simulink model "flightControlSystem"  (R2020a)
settings: Solver=ode3  StartTime=0  StopTime=TFinal  FixedStep=Ts  RelTol=1e-3  EnableMultiTasking=on
undefined symbols (not defined in the file): codertarget, Controller, DiscIntNeverNeededParam, Discrete, Estimator, g, gray, init, orient_ref, pos_ref, Sensors, Time, Ts, Vehicle
libraries: simulink x37, sharedtransform x3, ctrlSharedLib x2, visionstatistics x2, visiontransforms x2, sharedutil x1, visiontextngfix x1, visionanalysis x1, parrotlib x1
(part 2 of 2)

== system flightControlSystem/Control System/State Estimator/EstimatorXYPosition ==
  opticalFlow_datin : Inport
  controlModePosVSOrient_flagin : Inport  Port=2
  sensorIMU_datin : Inport  Port=3
  Z_estimin : Inport  Port=4
  dz_estimin : Inport  Port=5
  orient_estimin : Inport  Port=6
  EstimatorVelocity : Subsystem
  EstimatorXYPosition : Subsystem
  XY_estimout : Outport  VectorParamsAs1DForOutWhenUnconnected=off
  dxy_estimout : Outport  Port=2  VectorParamsAs1DForOutWhenUnconnected=off
  wires:
  EstimatorXYPosition/1(XY_estimout) -> XY_estimout/1
  dz_estimin/1 -> EstimatorXYPosition/4(dz_estimin)
  controlModePosVSOrient_flagin/1 -> EstimatorXYPosition/3(controlModePosVSOrient_flagin)
  Z_estimin/1 -> EstimatorVelocity/2(Z_estimin)
  sensorIMU_datin/1 -> EstimatorVelocity/3(sensorIMU_datin)
  opticalFlow_datin/1 -> EstimatorVelocity/1(opticalFlow_datin)
  EstimatorVelocity/1(dxy_estimout) -> dxy_estimout/1, EstimatorXYPosition/1(dxy_estimin)
  orient_estimin/1 -> EstimatorVelocity/4(orient_estimin), EstimatorXYPosition/2(orient_estimin)

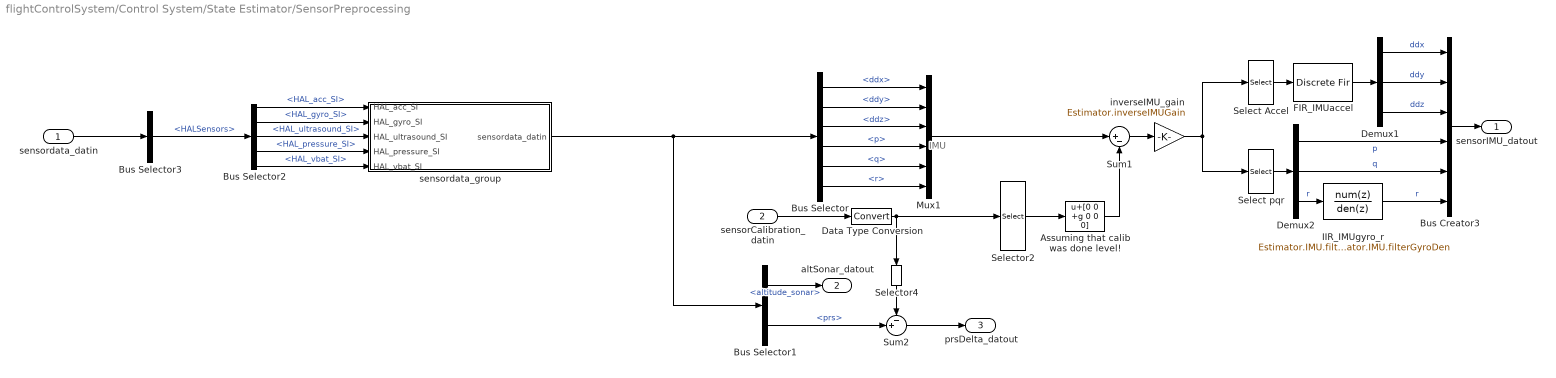
== system flightControlSystem/Control System/State Estimator/SensorPreprocessing ==
  note: IMU
  sensordata_datin : Inport
  sensorCalibration_datin : Inport  Port=2
  Assuming that calib was done level! : Bias  Bias=[0 0 +g 0 0 0]
  Bus Creator3 : BusCreator  Inputs=6
  Bus Selector : BusSelector  OutputSignals=ddx,ddy,ddz,p,q,r
  Bus Selector1 : BusSelector  OutputSignals=altitude_sonar,prs
  Bus Selector2 : BusSelector  OutputSignals=HAL_acc_SI,HAL_gyro_SI,HAL_ultrasound_SI,HAL_pressure_SI,HAL_vbat_SI
  Bus Selector3 : BusSelector  OutputSignals=HALSensors
  Data Type Conversion : DataTypeConversion
  Demux1 : Demux  Outputs=3
  Demux2 : Demux  Outputs=3
  FIR_IMUaccel : DiscreteFir  Coefficients=Estimator.IMU.filterAccel.Coefficients
  IIR_IMUgyro_r : DiscreteFilter  Numerator=Estimator.IMU.filterGyroNum  Denominator=Estimator.IMU.filterGyroDen
  Mux1 : Mux  Inputs=6
  Select Accel : Selector  InputPortWidth=6  IndexOptions=Index vector (dialog)  Indices=[1 2 3]  OutputSizes=1
  Select pqr : Selector  InputPortWidth=6  IndexOptions=Index vector (dialog)  Indices=[4 5 6]  OutputSizes=1
  Selector2 : Selector  InputPortWidth=8  IndexOptions=Index vector (dialog)  Indices=[1:6]  OutputSizes=1
  Selector4 : Selector  InputPortWidth=8  IndexOptions=Index vector (dialog)  Indices=[7]  OutputSizes=1
  Sum1 : Sum  Inputs=|+-
  Sum2 : Sum  Inputs=-+|
  inverseIMU_gain : Gain  Gain=Estimator.inverseIMUGain  ParamDataTypeStr=single  OutDataTypeStr=single
  sensordata_group : Subsystem
  sensorIMU_datout : Outport  VectorParamsAs1DForOutWhenUnconnected=off
  altSonar_datout : Outport  Port=2  VectorParamsAs1DForOutWhenUnconnected=off
  prsDelta_datout : Outport  Port=3  VectorParamsAs1DForOutWhenUnconnected=off
  wires:
  Select pqr/1 -> Demux2/1
  Assuming that calib was done level!/1 -> Sum1/2
  Mux1/1 -> Sum1/1
  Sum2/1 -> prsDelta_datout/1
  Bus Selector1/2 -> Sum2/2  "<prs>"
  Selector4/1 -> Sum2/1
  Bus Selector1/1 -> altSonar_datout/1  "<altitude_sonar>"
  Bus Selector/6 -> Mux1/6  "<r>"
  Bus Selector/5 -> Mux1/5  "<q>"
  Bus Selector/4 -> Mux1/4  "<p>"
  Bus Selector/3 -> Mux1/3  "<ddz>"
  Bus Selector/2 -> Mux1/2  "<ddy>"
  Bus Selector/1 -> Mux1/1  "<ddx>"
  sensorCalibration_datin/1 -> Data Type Conversion/1
  IIR_IMUgyro_r/1 -> Bus Creator3/6  "r"
  Demux2/3 -> IIR_IMUgyro_r/1  "r"
  FIR_IMUaccel/1 -> Demux1/1
  Select Accel/1 -> FIR_IMUaccel/1
  inverseIMU_gain/1 -> Select Accel/1, Select pqr/1
  Demux2/2 -> Bus Creator3/5  "q"
  Demux2/1 -> Bus Creator3/4  "p"
  Selector2/1 -> Assuming that calib was done level!/1
  Sum1/1 -> inverseIMU_gain/1
  Demux1/3 -> Bus Creator3/3  "ddz"
  Demux1/2 -> Bus Creator3/2  "ddy"
  Demux1/1 -> Bus Creator3/1  "ddx"
  Bus Creator3/1 -> sensorIMU_datout/1
  Data Type Conversion/1 -> Selector2/1, Selector4/1
  Bus Selector2/2 -> sensordata_group/2(HAL_gyro_SI)  "<HAL_gyro_SI>"
  Bus Selector2/4 -> sensordata_group/4(HAL_pressure_SI)  "<HAL_pressure_SI>"
  Bus Selector2/5 -> sensordata_group/5(HAL_vbat_SI)  "<HAL_vbat_SI>"
  Bus Selector2/3 -> sensordata_group/3(HAL_ultrasound_SI)  "<HAL_ultrasound_SI>"
  Bus Selector3/1 -> Bus Selector2/1  "<HALSensors>"
  sensordata_group/1(sensordata_datin) -> Bus Selector1/1, Bus Selector/1
  sensordata_datin/1 -> Bus Selector3/1
  Bus Selector2/1 -> sensordata_group/1(HAL_acc_SI)  "<HAL_acc_SI>"

== system flightControlSystem/Control System/State Estimator/Complementary Filter/If Action Subsystem ==
  rpy : Inport
  accel : Inport  Port=2
  Action Port : ActionPort  ActionPortLabel=if(u1 > 0)
  Demux : Demux  Outputs=3
  Demux1 : Demux  Outputs=3
  Divide : Product  Inputs=*/
  Gain : Gain  Gain=1-Estimator.gyroAngleUpdateAccWeight
  Gain1 : Gain  Gain=Estimator.gyroAngleUpdateAccWeight
  Gain2 : Gain  Gain=1/g
  Gain3 : Gain  Gain=Estimator.gyroAngleUpdateAccWeight
  Gain4 : Gain  Gain=1-Estimator.gyroAngleUpdateAccWeight
  Mux : Mux  Inputs=2
  Sum : Sum  Inputs=|++
  Sum1 : Sum  Inputs=|++
  Terminator1 : Terminator
  Trigonometric Function : Trigonometry  Operator=atan
  Trigonometric Function1 : Trigonometry  Operator=asin
  pitch,roll : Outport  VectorParamsAs1DForOutWhenUnconnected=off
  wires:
  accel/1 -> Demux/1
  Demux/2 -> Divide/1
  Demux/3 -> Divide/2
  Divide/1 -> Trigonometric Function/1
  Gain/1 -> Sum/1
  Trigonometric Function/1 -> Gain1/1
  Mux/1 -> pitch,roll/1
  Gain2/1 -> Trigonometric Function1/1
  Trigonometric Function1/1 -> Gain3/1
  Gain4/1 -> Sum1/1
  Gain3/1 -> Sum1/2
  Sum1/1 -> Mux/1
  Sum/1 -> Mux/2
  rpy/1 -> Demux1/1
  Demux1/1 -> Gain/1
  Demux1/2 -> Gain4/1
  Demux/1 -> Gain2/1
  Demux1/3 -> Terminator1/1
  Gain1/1 -> Sum/2

== system flightControlSystem/Control System/State Estimator/Complementary Filter/If Action Subsystem2 ==
  prin : Inport
  Action Port : ActionPort  ActionPortLabel=else
  prout : Outport  VectorParamsAs1DForOutWhenUnconnected=off
  wires:
  prin/1 -> prout/1

== system flightControlSystem/Control System/State Estimator/Complementary Filter/Wbe ==
  rpy : Inport  OutDataTypeStr=single
  Constant : Constant  Value=single(0)
  Create 3x3 Matrix : sharedutil/Create 3x3 Matrix  aMode=aMode
      settings: SourceProductBaseCode=AE,PW,MT,VE,VP
  Divide : Product  Inputs=*/
  Gain : Gain  Gain=-1
  Product{1..4} (4 alike) : Product
  Selector : Selector  InputPortWidth=3  IndexOptions=Index vector (dialog)  Indices=[1]  OutputSizes=1
  Selector1 : Selector  InputPortWidth=3  IndexOptions=Index vector (dialog)  Indices=[1]  OutputSizes=1
  Selector2 : Selector  InputPortWidth=3  IndexOptions=Index vector (dialog)  Indices=[2]  OutputSizes=1
  Selector3 : Selector  InputPortWidth=3  IndexOptions=Index vector (dialog)  Indices=[2]  OutputSizes=1
  Trigonometric Function : Trigonometry  Operator=sincos
  Wbe : Outport  VectorParamsAs1DForOutWhenUnconnected=off
  wires:
  Create 3x3 Matrix/1 -> Divide/1
  Product3/1 -> Create 3x3 Matrix/8
  Trigonometric Function/2 -> Selector1/1, Selector2/1
  Selector3/1 -> Product4/2, Product3/2
  Selector1/1 -> Product4/1, Product1/1, Create 3x3 Matrix/3
  Trigonometric Function/1 -> Selector3/1, Selector/1
  Product1/1 -> Create 3x3 Matrix/5
  Product2/1 -> Create 3x3 Matrix/6
  Selector2/1 -> Divide/2, Create 3x3 Matrix/7, Product2/1, Product1/2
  Gain/1 -> Product2/2
  Product4/1 -> Create 3x3 Matrix/9
  Constant/1 -> Create 3x3 Matrix/4, Create 3x3 Matrix/1
  Divide/1 -> Wbe/1
  rpy/1 -> Trigonometric Function/1
  Selector/1 -> Product3/1, Gain/1, Create 3x3 Matrix/2

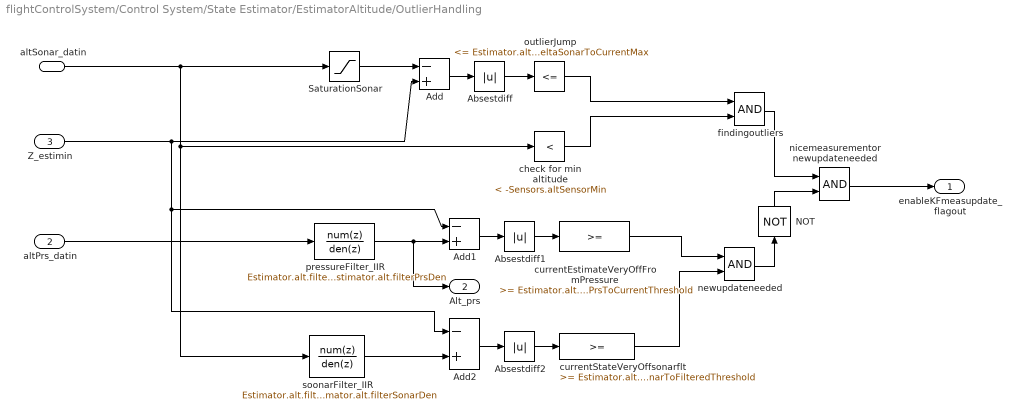
== system flightControlSystem/Control System/State Estimator/EstimatorAltitude/OutlierHandling ==
  altSonar_datin : Inport
  altPrs_datin : Inport  Port=2
  Z_estimin : Inport  Port=3
  Absestdiff : Abs
  Absestdiff1 : Abs
  Absestdiff2 : Abs
  Add : Sum  Inputs=-+
  Add1 : Sum  Inputs=-+
  Add2 : Sum  Inputs=-+
  NOT : Logic  Operator=NOT  IconShape=distinctive  AllPortsSameDT=off  OutDataTypeStr=boolean
  SaturationSonar : Saturate  UpperLimit=-Sensors.altSensorMin  LowerLimit=-inf
  check for min altitude : simulink/Logic and Bit Operations/Compare To Constant  relop=<  const=-Sensors.altSensorMin  OutDataTypeStr=boolean
  currentEstimateVeryOffFromPressure : simulink/Logic and Bit Operations/Compare To Constant  relop=>=  const=Estimator.alt.deltaPrsToCurrentThreshold  OutDataTypeStr=boolean
  currentStateVeryOffsonarflt : simulink/Logic and Bit Operations/Compare To Constant  relop=>=  const=Estimator.alt.deltaSonarToFilteredThreshold  OutDataTypeStr=boolean
  findingoutliers : Logic  AllPortsSameDT=off  OutDataTypeStr=boolean
  newupdateneeded : Logic  AllPortsSameDT=off  OutDataTypeStr=boolean
  nicemeasurementor newupdateneeded : Logic  AllPortsSameDT=off  OutDataTypeStr=boolean
  outlierJump : simulink/Logic and Bit Operations/Compare To Constant  relop=<=  const=Estimator.alt.deltaSonarToCurrentMax  OutDataTypeStr=boolean
  pressureFilter_IIR : DiscreteFilter  Numerator=Estimator.alt.filterPrsNum  Denominator=Estimator.alt.filterPrsDen
  soonarFilter_IIR : DiscreteFilter  Numerator=Estimator.alt.filterSonarNum  Denominator=Estimator.alt.filterSonarDen
  enableKFmeasupdate_flagout : Outport  VectorParamsAs1DForOutWhenUnconnected=off
  Alt_prs : Outport  Port=2  VectorParamsAs1DForOutWhenUnconnected=off
  wires:
  Add1/1 -> Absestdiff1/1
  nicemeasurementor newupdateneeded/1 -> enableKFmeasupdate_flagout/1
  findingoutliers/1 -> nicemeasurementor newupdateneeded/1
  check for min altitude/1 -> findingoutliers/2
  outlierJump/1 -> findingoutliers/1
  SaturationSonar/1 -> Add/1
  Absestdiff/1 -> outlierJump/1
  Add/1 -> Absestdiff/1
  newupdateneeded/1 -> NOT/1
  Absestdiff2/1 -> currentStateVeryOffsonarflt/1
  altSonar_datin/1 -> SaturationSonar/1, soonarFilter_IIR/1, check for min altitude/1
  currentEstimateVeryOffFromPressure/1 -> newupdateneeded/1
  Z_estimin/1 -> Add1/1, Add2/1, Add/2
  Add2/1 -> Absestdiff2/1
  currentStateVeryOffsonarflt/1 -> newupdateneeded/2
  pressureFilter_IIR/1 -> Alt_prs/1, Add1/2
  altPrs_datin/1 -> pressureFilter_IIR/1
  soonarFilter_IIR/1 -> Add2/2
  Absestdiff1/1 -> currentEstimateVeryOffFromPressure/1
  NOT/1 -> nicemeasurementor newupdateneeded/2

== system flightControlSystem/Control System/State Estimator/EstimatorXYPosition/EstimatorVelocity ==
  opticalFlow_datin : Inport
  Z_estimin : Inport  Port=2  SampleTime=Ts
  sensorIMU_datin : Inport  Port=3
  orient_estimin : Inport  Port=4
  " " : Product  Inputs=**
  AccelerationHandling : Subsystem
  Compare To Constant : simulink/Logic and Bit Operations/Compare To Constant  relop=<  const=200*4  OutDataTypeStr=boolean
  Counter Free-Running : simulink/Sources/Counter Free-Running  NumBits=32  tsamp=-1
  DataHandling : Subsystem
  Delay : Delay  DelayLength=1  InitialCondition=0
  Gain : Gain  Gain=-1
  KalmanFilter_dxdy : ctrlSharedLib/Kalman Filter  TimeDomain=Discrete-Time  UseCurrentEstimator=on  ModelSource=Individual A, B, C, D matrices  ModelSourceVariable=ss(0.95,1,1,0,1)  A=eye(2)  B=Ts*eye(2)  C=eye(2)  D=0  NumberOfStates=1  NumberOfInputs=1  NumberOfOutputs=1  InitialEstimateSource=Dialog  X0=0  P0=10  UseK=off  UseGH=on  NumberOfProcessNoiseInputs=1  G=Estimator.pos.kfVelo.G  TimeInvariantG=on  H=Estimator.pos.kfVelo.H  TimeInvariantH=on  Q=Estimator.pos.kfVelo.Q  TimeInvariantQ=on  R=Estimator.pos.kfVelo.R  TimeInvariantR=on  N=Estimator.pos.kfVelo.N  TimeInvariantN=on  AddInputPort=on  AddEnablePort=on  OutputEstimatedY=off  OutputP=off  Ts=-1
  Select dxy : Selector  InputPortWidth=3  IndexOptions=Index vector (dialog)  Indices=[1 2]  OutputSizes=1
  Switch : Switch  Criteria=u2 > Threshold
  Z_estimin1 : InportShadow  Port=2  SampleTime=Ts
  opticalFlowErrorCorrect : Gain  Gain=1.15
  dxy_estimout : Outport  VectorParamsAs1DForOutWhenUnconnected=off
  wires:
  Delay/1 -> DataHandling/5(dxyOF_datin)
  Z_estimin/1 -> DataHandling/1(Z_estimin), AccelerationHandling/4(Z_estimin)
  KalmanFilter_dxdy/1 -> dxy_estimout/1, Delay/1
  sensorIMU_datin/1 -> AccelerationHandling/2(sensorIMU_datin), DataHandling/3(sensorIMU_datin)
  orient_estimin/1 -> AccelerationHandling/3(orient_estimin), DataHandling/2(orient_estimin)
  Select dxy/1 -> KalmanFilter_dxdy/2, AccelerationHandling/1(dxy_estimin), DataHandling/4(dxy_estimin)
  AccelerationHandling/1(acceleration_world) -> KalmanFilter_dxdy/1
  DataHandling/1(enable_flag) -> KalmanFilter_dxdy/3
  Switch/1 -> Select dxy/1
  " "/1 -> opticalFlowErrorCorrect/1
  Gain/1 -> " "/2
  opticalFlowErrorCorrect/1 -> Switch/3
  Compare To Constant/1 -> Switch/2
  opticalFlow_datin/1 -> " "/1, Switch/1
  Z_estimin1/1 -> Gain/1
  Counter Free-Running/1 -> Compare To Constant/1

== system flightControlSystem/Control System/State Estimator/EstimatorXYPosition/EstimatorXYPosition ==
  note: Switching from orientationControl to Position
      | control reset the current world position estimate
      | (happens when using no markers)
  dxy_estimin : Inport
  orient_estimin : Inport  Port=2  SampleTime=Ts
  controlModePosVSOrient_flagin : Inport  Port=3
  dz_estimin : Inport  Port=4
  Math Function : Math  Operator=transpose  SignedPower=on  SaturateOnIntegerOverflow=on
  Mux2 : Mux  Inputs=2
  Product : Product  Multiplication=Matrix(*)
  Rotation Angles to Direction Cosine Matrix : sharedtransform/Rotation Angles to Direction Cosine Matrix  rotationOrder=ZYX  aMode=aMode
      settings: SourceProductBaseCode=AE,PW,MT,VE,VP
  SelectdXY : Selector  InputPortWidth=3  IndexOptions=Index vector (dialog)  Indices=[1 2]  OutputSizes=1
  SimplyIntegrateVelocity : DiscreteIntegrator  ExternalReset=rising  SampleTime=Ts  ICPrevOutput=DiscIntNeverNeededParam  ICPrevScaledInput=DiscIntNeverNeededParam
  XY_estimout : Outport  VectorParamsAs1DForOutWhenUnconnected=off
  wires:
  controlModePosVSOrient_flagin/1 -> SimplyIntegrateVelocity/2
  Product/1 -> SelectdXY/1
  Mux2/1 -> Product/2
  dz_estimin/1 -> Mux2/2
  SimplyIntegrateVelocity/1 -> XY_estimout/1
  dxy_estimin/1 -> Mux2/1
  orient_estimin/1 -> Rotation Angles to Direction Cosine Matrix/1
  Rotation Angles to Direction Cosine Matrix/1 -> Math Function/1
  SelectdXY/1 -> SimplyIntegrateVelocity/1
  Math Function/1 -> Product/1

== system flightControlSystem/Control System/State Estimator/SensorPreprocessing/sensordata_group ==
  HAL_acc_SI : Inport  OutDataTypeStr=Bus: HAL_acc_SI_t
  HAL_gyro_SI : Inport  Port=2  OutDataTypeStr=Bus: HAL_gyro_SI_t
  HAL_ultrasound_SI : Inport  Port=3  OutDataTypeStr=Bus: HAL_ultrasound_SI_t
  HAL_pressure_SI : Inport  Port=4  OutDataTypeStr=Bus: HAL_pressure_SI_t
  HAL_vbat_SI : Inport  Port=5  OutDataTypeStr=Bus: HAL_vbat_SI_t
  Bus Selector1 : BusSelector  OutputSignals=vbat_V,vbat_percentage
  Bus Selector3 : BusSelector  OutputSignals=x,y,z
  Bus Selector4 : BusSelector  OutputSignals=x,y,z
  Bus Selector5 : BusSelector  OutputSignals=altitude
  Bus Selector6 : BusSelector  OutputSignals=pressure
  Out Bus Element : Outport  VectorParamsAs1DForOutWhenUnconnected=off  PortName=sensordata_datin  Element=ddx
  Out Bus Element1 : Outport  VectorParamsAs1DForOutWhenUnconnected=off  PortName=sensordata_datin  Element=ddy
  Out Bus Element2 : Outport  VectorParamsAs1DForOutWhenUnconnected=off  PortName=sensordata_datin  Element=ddz
  Out Bus Element3 : Outport  VectorParamsAs1DForOutWhenUnconnected=off  PortName=sensordata_datin  Element=p
  Out Bus Element4 : Outport  VectorParamsAs1DForOutWhenUnconnected=off  PortName=sensordata_datin  Element=q
  Out Bus Element5 : Outport  VectorParamsAs1DForOutWhenUnconnected=off  PortName=sensordata_datin  Element=r
  Out Bus Element6 : Outport  VectorParamsAs1DForOutWhenUnconnected=off  PortName=sensordata_datin  Element=altitude_sonar
  Out Bus Element7 : Outport  VectorParamsAs1DForOutWhenUnconnected=off  PortName=sensordata_datin  Element=prs
  Out Bus Element8 : Outport  VectorParamsAs1DForOutWhenUnconnected=off  PortName=sensordata_datin  Element=vbat_V
  Out Bus Element9 : Outport  VectorParamsAs1DForOutWhenUnconnected=off  PortName=sensordata_datin  Element=vbat_percentage
  wires:
  HAL_gyro_SI/1 -> Bus Selector4/1
  HAL_acc_SI/1 -> Bus Selector3/1
  HAL_pressure_SI/1 -> Bus Selector6/1
  HAL_ultrasound_SI/1 -> Bus Selector5/1
  Bus Selector4/1 -> Out Bus Element3/1  "<x>"
  Bus Selector3/3 -> Out Bus Element2/1  "<z>"
  Bus Selector4/3 -> Out Bus Element5/1  "<z>"
  Bus Selector5/1 -> Out Bus Element6/1  "<altitude>"
  Bus Selector6/1 -> Out Bus Element7/1  "<pressure>"
  Bus Selector4/2 -> Out Bus Element4/1  "<y>"
  Bus Selector3/1 -> Out Bus Element/1  "<x>"
  Bus Selector3/2 -> Out Bus Element1/1  "<y>"
  Bus Selector1/1 -> Out Bus Element8/1  "<vbat_V>"
  HAL_vbat_SI/1 -> Bus Selector1/1
  Bus Selector1/2 -> Out Bus Element9/1  "<vbat_percentage>"

== system flightControlSystem/Control System/State Estimator/EstimatorXYPosition/EstimatorVelocity/AccelerationHandling ==
  dxy_estimin : Inport
  sensorIMU_datin : Inport  Port=2
  orient_estimin : Inport  Port=3
  Z_estimin : Inport  Port=4
  Add : Sum  Inputs=-+
  Bus Selector1 : BusSelector  OutputSignals=ddx,ddy,ddz
  Deactivate Acceleration If OF is not used due to low altitude : simulink/Logic and Bit Operations/Compare To Constant  relop=<=  const=Estimator.pos.opticalFlowZMax  OutDataTypeStr=boolean
  Logical Operator : Logic  Operator=OR  AllPortsSameDT=off  OutDataTypeStr=boolean
  Mux6 : Mux  Inputs=3
  Product : Product  Inputs=3
  Product1 : Product  Multiplication=Matrix(*)
  Rotation Angles to Direction Cosine Matrix : sharedtransform/Rotation Angles to Direction Cosine Matrix  rotationOrder=ZYX  aMode=aMode
      settings: SourceProductBaseCode=AE,PW,MT,VE,VP
  SelectPlanarddxy : Selector  InputPortWidth=3  IndexOptions=Index vector (dialog)  Indices=[1 2]  OutputSizes=1
  Selector : Selector  InputPortWidth=2  IndexOptions=Index vector (dialog)  Indices=1  OutputSizes=1
  Selector1 : Selector  InputPortWidth=2  IndexOptions=Index vector (dialog)  Indices=2  OutputSizes=1
  do not use acc if optical flow never available (Note OF@60Hz but ZOH to 200!) : simulink/Logic and Bit Operations/Compare To Constant  relop=~=  const=0  OutDataTypeStr=boolean
  do not use acc if optical flow never available (Note OF@60Hz but ZOH to 200!)1 : simulink/Logic and Bit Operations/Compare To Constant  relop=~=  const=0  OutDataTypeStr=boolean
  gainaccinput : Gain  Gain=Estimator.pos.accelerationInputGain  OutDataTypeStr=single
  gravity : Constant  Value=[0 0 -g]
  acceleration_world : Outport  OutDataTypeStr=single  VectorParamsAs1DForOutWhenUnconnected=off
  wires:
  do not use acc if optical flow never available (Note OF@60Hz but ZOH to 200!)1/1 -> Logical Operator/2
  do not use acc if optical flow never available (Note OF@60Hz but ZOH to 200!)/1 -> Logical Operator/1
  Logical Operator/1 -> Product/1
  Selector1/1 -> do not use acc if optical flow never available (Note OF@60Hz but ZOH to 200!)1/1
  Selector/1 -> do not use acc if optical flow never available (Note OF@60Hz but ZOH to 200!)/1
  dxy_estimin/1 -> Selector1/1, Selector/1
  Product/1 -> acceleration_world/1
  Deactivate Acceleration If OF is not used due to low altitude/1 -> Product/3
  Z_estimin/1 -> Deactivate Acceleration If OF is not used due to low altitude/1
  Add/1 -> SelectPlanarddxy/1
  Product1/1 -> Add/1
  gravity/1 -> Product1/2
  gainaccinput/1 -> Product/2
  SelectPlanarddxy/1 -> gainaccinput/1
  Bus Selector1/3 -> Mux6/3  "<ddz>"
  Bus Selector1/1 -> Mux6/1  "<ddx>"
  sensorIMU_datin/1 -> Bus Selector1/1
  Mux6/1 -> Add/2
  Bus Selector1/2 -> Mux6/2  "<ddy>"
  orient_estimin/1 -> Rotation Angles to Direction Cosine Matrix/1
  Rotation Angles to Direction Cosine Matrix/1 -> Product1/1

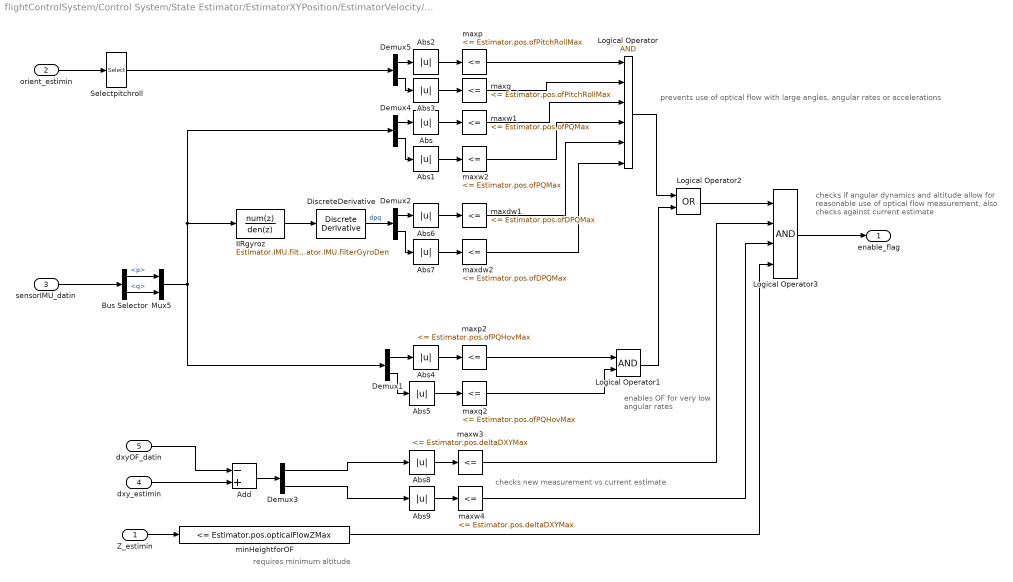
== system flightControlSystem/Control System/State Estimator/EstimatorXYPosition/EstimatorVelocity/DataHandling ==
  note: prevents use of optical flow with large angles, angular rates or accelerations
  note: enables OF for very
      | low angular rates
  note: checks if angular dynamics and altitude allow for
      | reasonable use of optical flow measurement,
      | also checks against current estimate
  note: checks new measurement vs current estimate
  note: requires minimum altitude
  Z_estimin : Inport
  orient_estimin : Inport  Port=2
  sensorIMU_datin : Inport  Port=3
  dxy_estimin : Inport  Port=4
  dxyOF_datin : Inport  Port=5
  Abs{,1..9} (10 alike) : Abs
  Add : Sum  Inputs=-+
  Bus Selector : BusSelector  OutputSignals=p,q
  Demux{1..5} (5 alike) : Demux  Outputs=2
  DiscreteDerivative : simulink/Discrete/Discrete Derivative  gainval=1.0  ICPrevScaledInput=0.0  OutMin=[]  OutMax=[]  OutDataType=fixdt(1, 16)  OutScaling=2^-10  DoSatur=off
  IIRgyroz : DiscreteFilter  Numerator=Estimator.IMU.filterGyroNum  Denominator=Estimator.IMU.filterGyroDen
  Logical Operator : Logic  Inputs=6  AllPortsSameDT=off  OutDataTypeStr=boolean
  Logical Operator1 : Logic  AllPortsSameDT=off  OutDataTypeStr=boolean
  Logical Operator2 : Logic  Operator=OR  AllPortsSameDT=off  OutDataTypeStr=boolean
  Logical Operator3 : Logic  Inputs=4  AllPortsSameDT=off  OutDataTypeStr=boolean
  Mux5 : Mux  Inputs=2
  Selectpitchroll : Selector  InputPortWidth=3  IndexOptions=Index vector (dialog)  Indices=[2 3]  OutputSizes=1
  maxdw1 : simulink/Logic and Bit Operations/Compare To Constant  relop=<=  const=Estimator.pos.ofDPQMax  OutDataTypeStr=boolean
  maxdw2 : simulink/Logic and Bit Operations/Compare To Constant  relop=<=  const=Estimator.pos.ofDPQMax  OutDataTypeStr=boolean
  maxp : simulink/Logic and Bit Operations/Compare To Constant  relop=<=  const=Estimator.pos.ofPitchRollMax  OutDataTypeStr=boolean
  maxp2 : simulink/Logic and Bit Operations/Compare To Constant  relop=<=  const=Estimator.pos.ofPQHovMax  OutDataTypeStr=boolean
  maxq : simulink/Logic and Bit Operations/Compare To Constant  relop=<=  const=Estimator.pos.ofPitchRollMax  OutDataTypeStr=boolean
  maxq2 : simulink/Logic and Bit Operations/Compare To Constant  relop=<=  const=Estimator.pos.ofPQHovMax  OutDataTypeStr=boolean
  maxw1 : simulink/Logic and Bit Operations/Compare To Constant  relop=<=  const=Estimator.pos.ofPQMax  OutDataTypeStr=boolean
  maxw2 : simulink/Logic and Bit Operations/Compare To Constant  relop=<=  const=Estimator.pos.ofPQMax  OutDataTypeStr=boolean
  maxw3 : simulink/Logic and Bit Operations/Compare To Constant  relop=<=  const=Estimator.pos.deltaDXYMax  OutDataTypeStr=boolean
  maxw4 : simulink/Logic and Bit Operations/Compare To Constant  relop=<=  const=Estimator.pos.deltaDXYMax  OutDataTypeStr=boolean
  minHeightforOF : simulink/Logic and Bit Operations/Compare To Constant  relop=<=  const=Estimator.pos.opticalFlowZMax  OutDataTypeStr=boolean
  enable_flag : Outport  VectorParamsAs1DForOutWhenUnconnected=off
  wires:
  minHeightforOF/1 -> Logical Operator3/4
  IIRgyroz/1 -> DiscreteDerivative/1
  Mux5/1 -> Demux1/1, IIRgyroz/1, Demux4/1
  maxw4/1 -> Logical Operator3/3
  maxw3/1 -> Logical Operator3/2
  dxyOF_datin/1 -> Add/1
  Demux3/2 -> Abs9/1
  Demux3/1 -> Abs8/1
  dxy_estimin/1 -> Add/2
  Add/1 -> Demux3/1
  Abs9/1 -> maxw4/1
  Abs8/1 -> maxw3/1
  Logical Operator2/1 -> Logical Operator3/1
  Logical Operator3/1 -> enable_flag/1
  DiscreteDerivative/1 -> Demux2/1  "dpq"
  Demux2/2 -> Abs7/1
  Demux2/1 -> Abs6/1
  Abs7/1 -> maxdw2/1
  Abs6/1 -> maxdw1/1
  Logical Operator1/1 -> Logical Operator2/2
  Demux1/2 -> Abs5/1
  Demux1/1 -> Abs4/1
  Abs5/1 -> maxq2/1
  Abs4/1 -> maxp2/1
  Abs3/1 -> maxq/1
  Abs2/1 -> maxp/1
  Demux4/2 -> Abs1/1
  Demux4/1 -> Abs/1
  Abs1/1 -> maxw2/1
  Abs/1 -> maxw1/1
  Z_estimin/1 -> minHeightforOF/1
  Logical Operator/1 -> Logical Operator2/1
  maxw1/1 -> Logical Operator/3
  Bus Selector/1 -> Mux5/1  "<p>"
  Selectpitchroll/1 -> Demux5/1
  sensorIMU_datin/1 -> Bus Selector/1
  maxq2/1 -> Logical Operator1/2
  Bus Selector/2 -> Mux5/2  "<q>"
  maxp/1 -> Logical Operator/1
  maxw2/1 -> Logical Operator/4
  orient_estimin/1 -> Selectpitchroll/1
  maxdw1/1 -> Logical Operator/5
  maxdw2/1 -> Logical Operator/6
  maxq/1 -> Logical Operator/2
  Demux5/1 -> Abs2/1
  Demux5/2 -> Abs3/1
  maxp2/1 -> Logical Operator1/1

== matlab function flightControlSystem/Image Processing System/LINE ALGORITHM/Path Centroid Finder ==
  data: pic input; XYCoOrd output; XYPair input

function XYCoOrd = Centroid_Finder(pic,XYPair)
picHEIGHT = size(pic,1); picWIDTH = size(pic,2);
XYCoOrd = -1*ones(2,1); %Default NULL detection
if (isempty(XYPair))%If no bounding points, return NULL
    return;
end
%Find number of HIGH pixels
HIGH_x = 0; HIGH_y = 0; HIGH_pix = 0;
for y = 1:picHEIGHT
    for x = 1:picWIDTH
        if (pic(y,x))
            HIGH_pix = HIGH_pix+1;
            HIGH_x = HIGH_x+x;
            HIGH_y = HIGH_y+y;
        end
    end
end
%Default mode is to continue along path
XYCoOrd(1) = pi/2; % theta
XYCoOrd(2) = 0;    % rho
if (HIGH_pix ~= 0)
    XYCoOrd(1) = HIGH_x/HIGH_pix; % centroid pixel x
    XYCoOrd(2) = HIGH_y/HIGH_pix; % centroid pixel y
end
end

== matlab function flightControlSystem/Image Processing System/LINE ALGORITHM/XYtoHesse ==
  data: img input; XYCoOrd input; Theta output; Rho output
function [Theta, Rho] = XYtoHesse(img,XYCoOrd)
if XYCoOrd==-1*ones(2,1)
    Theta=-1; Rho=-1; %Nothing Detected
    return;
end
X = size(img,1); Y = size(img,2);
%Move to origin
XYCoOrd(1) = XYCoOrd(1) - Y/2;
XYCoOrd(2) = XYCoOrd(2) - X/2;
%Convert from Cartesian to Hesse
Theta = mod(-atan2(XYCoOrd(2),XYCoOrd(1)),2*pi);
Rho = sqrt(XYCoOrd(1)^2 + XYCoOrd(2)^2);
%%BAAAAAA
end

== matlab function flightControlSystem/Control System/Path Planning/Linear Path/XY Trajectory ==
  data: LineAngle input; Centroid input; FlyMode input; Gain input; Speed input; dx output double; prev_Hough input; dy output double; Hough_Angle output; prev_Centroid input; Centroid_Angle output
function [dx, dy, Hough_Angle, Centroid_Angle] = XY_Traj(LineAngle,Centroid, FlyMode,Gain,Speed ,prev_Hough, prev_Centroid)
Hough_Angle = prev_Hough;
Centroid_Angle = prev_Centroid;
minError = 2*pi;
%%
%For each coordline
for i = 1:8
    %If no line detected
    if (LineAngle(i) == -1)
        continue
    end
    %Detect whether trajectory needs alteration
    Angle_Error = Angle_diff(LineAngle(i),prev_Hough);
    %if traj requires change (less than a full 180 so no backwards action)
    if Angle_Error < minError && Angle_Error < deg2rad(170) %~10deg error bar
        Hough_Angle = LineAngle(i);
        minError = Angle_Error;
    end
end

%%
%Move towards path/circle centroid
Centroid_Angle = Centroid(1);
Centroid_Step = Speed*Gain*Centroid(2);
dx = Centroid_Step*sin(Centroid_Angle);
dy = Centroid_Step*cos(Centroid_Angle);

%%
%If in flight mode add increment to continue flying along Hough Line
if (FlyMode == 1)
    dx = dx + Speed*sin(Hough_Angle);
    dy = dy + Speed*cos(Hough_Angle);
end
end
%%
function Angle_Error = Angle_diff(Phi, Theta)
Upper = max(Phi,Theta);
Lower = min(Phi,Theta);
Angle_Error = min(Upper-Lower, Lower+2*pi-Upper);
end

== stateflow chart flightControlSystem/Control System/Path Planning/Linear Path/Z Trajectory ==
  state Fly
    entry:
    FlyMode = prev_Mode;
    z = Z_hover;
    during:
    z = double(prev_z);
  state LandMode
    entry:
    FlyMode = 0;
  state Descent
    z = double(prev_z+Z_increment);
  (default) -> Fly
  Fly -> LandMode : [(CircleCentroid(2) ~= -1 )]
  LandMode -> Fly [order 2]
  LandMode -> Descent [order 1] : [(CircleCentroid(2) < Land_Dist)]
  data: CircleCentroid input; Land_Dist input; Z_hover input; Z_increment input; prev_Mode input; prev_z input; z output; FlyMode output

== stateflow chart flightControlSystem/Control System/Path Planning/Chart3 ==
  state HOVER
    entry:
    pitch=0;
  state FORWARDpitch
    during:
    pitch=pitch+500000000000000;
  (default) -> HOVER
  HOVER -> FORWARDpitch
  data: pitch output single

== matlab function flightControlSystem/Image Processing System/Circle Detection/XYtoHesse ==
  data: img input; XYCoOrd input; Theta output; Rho output
function [Theta, Rho] = XYtoHesse(img,XYCoOrd)
X = size(img,1); Y = size(img,2);
%Move to origin
XYCoOrd(1) = XYCoOrd(1) - Y/2;
XYCoOrd(2) = XYCoOrd(2) - X/2;
%Convert from Cartesian to Hesse
Theta = mod(-atan2(XYCoOrd(2),XYCoOrd(1)),2*pi);
Rho = sqrt(XYCoOrd(1)^2 + XYCoOrd(2)^2);
end

== matlab function flightControlSystem/Image Processing System/LINE ALGORITHM/Line Angle Finder ==
  data: pic input; Angles output; XYPair input; ErrorBar input
function Angles = Angle_Finder(pic,XYPair,ErrorBar)
Lines = 4;% Number of lines we want
Angles = -1*ones(8,1); %one column vector for angles

picHEIGHT = size(pic,1); picWIDTH = size(pic,2);
XYPair = [XYPair(:,[1 2]); XYPair(:,[3 4])]; %rearrange into coordinate pairs
assert(ErrorBar<100);
ErrorBar=int32(linspace(-ErrorBar,ErrorBar,ErrorBar*2-1));

for i = 1:size(XYPair,1) %For each Boundary CoOrdinate
    CoOrd = XYPair(i,:);
    if (CoOrd(1) == 0 && CoOrd(2) == 0)
        continue;
    end
    %Denote region for detection of bounding point
    Xpix = ErrorBar+CoOrd(1);           Ypix = ErrorBar+CoOrd(2);
    %Correct for the given pixel range extending below/beyond image border
    Xpix(Xpix<1) = 1;                   Ypix(Ypix<1) = 1;
    Xpix(Xpix>picWIDTH) = picWIDTH;     Ypix(Ypix>picHEIGHT) = picHEIGHT;
    
    %For any HIGH value within given pixel range
    if any(any(       pic(Ypix,Xpix)      ))
        if (i <= Lines)
            %Define Angle between the current coordinate and its partner 
            Angles(i) = -atan2(double(XYPair(i,2)-XYPair(i+Lines,2)),...
                double(XYPair(i,1)-XYPair(i+Lines,1)));
        else
            Angles(i) = -atan2(double(XYPair(i,2)-XYPair(i-Lines,2)),...
                double(XYPair(i,1)-XYPair(i-Lines,1)));
        end
        Angles(i) = mod(Angles(i),2*pi);%Scale to within boundaries
    else
        Angles(i) = -1; %No bounding points can be mapped within range
    end
end
end
